simulink model "hcu_main_dspace"  (Simulink 8.2)
settings: Solver=FixedStepDiscrete  StartTime=0.0  StopTime=Inf  FixedStep=0.005  RelTol=1e-3
PostLoadFcn:
  | , if any(exist('dsrtsu_mdlpostloadfcn', 'file') == [2, 3, 6]), try dsrtsu_mdlpostloadfcn('Execute', bdroot); catch fprintf('Error in PostLoadFcn (dsrtsu_mdlpostloadfcn) for model "%s":\n %s\n', bdroot, lasterr); end, end,
values from neighbouring files (symbols this model uses):
  C_TASK_5MS_S = (	C_TICK_TIME_S      	)    [hcu_local_hdr.m]
  ENUM_GEARPOSN_1ST = uint8(  1  )    [hcu_local_hdr.m]
  ENUM_GEARPOSN_2ND = uint8(  2  )    [hcu_local_hdr.m]
  ENUM_GEARPOSN_3RD = uint8(  3  )    [hcu_local_hdr.m]
  ENUM_GEARPOSN_4TH = uint8(  4  )    [hcu_local_hdr.m]
  ENUM_GEARPOSN_5TH = uint8(  5  )    [hcu_local_hdr.m]
  ENUM_GEARPOSN_6TH = uint8(  6  )    [hcu_local_hdr.m]
  ENUM_GEARPOSN_R = uint8(  7  )    [hcu_local_hdr.m]
undefined symbols (not defined in the file or in its folder): rticanmm_blockfcn, rticanmm_initfcn
libraries: rtimmsu_dsrtlib x3, simulink x2, hal x2, app x1, rtiethernetudplib x1, inp x1, outp x1, hcu_lib x1
(part 2 of 4)

== system hcu_main_dspace/RTICANMM MainBlock1 ==
  TXData : Inport
  ModelClose : Subsystem  mask(RTICANMMModelClose){}
  TRC Exclusion : rtimmsu_dsrtlib/TRC Exclusion
  TXINselector1 : BusSelector  OutputSignals=ADAS1.ADAS1_Checksum,ADAS1.ADAS1_LifeCount,ADAS1.ADAS_StrTqReq_A,ADAS1.ADAS_StrAngReq_A,ADAS1.ADAS_EPSMode,ADAS1.ADAS_StrTqReqProt,ADAS1.ADAS_StrTqReq,ADAS1.ADAS_StrAngReqProt,ADAS1.ADAS_StrAngReq,ADAS2.ADAS2_Checksum,ADAS2.ADAS2_LifeCount,ADAS2.ADAS_VehHoldReq,ADAS2.ADAS_BrakePrefillReq_A,ADAS2.ADAS_BrakePrefillReq,ADAS2.ADAS_AEBReq_A,ADAS2.ADAS_AEBReq,ADAS2.ADAS_ForceIdle_A,ADAS2.ADAS_DecReq_Prot,ADAS2.ADAS_DecReq,ADAS2.ADAS_DecReq_A,ADAS2.ADAS_TqReq_A,ADAS2.ADAS_ForceIdle,ADAS2.ADAS_TqReqProt,ADAS2.ADAS_TqReq,ADAS3.ADAS3_Checksum,ADAS3.ADAS3_LifeCount,ADAS3.ForceLowBeam,ADAS3.LeftTurnLightReq,ADAS3.RightTurnLightReq,ADAS3.HazardWarningReq,ADAS3.ADAS_MIL,ADAS3.RampDownEnable,ADAS3.RampDownTime,ADAS3.ADAS_ShftPosnReq_A,ADAS3.ADAS_ShftPosnReq,ADAS3.ADAS_VehSpdLim_A,ADAS3.ADAS_GearPosnReq_A,ADAS3.ADAS_GearPosnReq,ADAS3.ADAS_VehSpdLim,ADAS4.ADASFaultWarningReq,ADAS4.HapticWarningReq,ADAS4.ADAS_APSEnable,ADAS4.ADAS_PilotMode,ADAS4.ADAS_IGSAStatus,ADAS4.ADAS_LFCMode,ADAS4.ADAS_MAPPStatus,ADAS4.ADAS_MAPAStatus,ADAS4.ADAS_LCSStatus,ADAS4.ADAS_LFCStatus,ADAS4.ADAS_LKAStatus,ADAS4.ADAS_ACCStatus,ADAS4.ADAS_FCWStatus,ADAS4.ADAS_AEBStatus,ADAS4.MAPPHMIWarningReq,ADAS4.MAPAHMIWarningReq,ADAS4.LCSHMIWarningReq,ADAS4.LFCHMIWarningReq,ADAS4.LKAHMIWarningReq,ADAS4.IGSAHMIWarningReq,ADAS4.AEBHMIWarningReq,ADAS4.ACCHMIWarningReq,ADAS4.FCWHMIWarningReq,ADAS5.ADAS_FaultMode,ADAS5.ADAS_LaneModeR,ADAS5.ADAS_LaneModeL,ADAS5.SeleTimeGapLvl,ADAS5.SetTimeGapLvl,ADAS5.IGSASetSpeed,ADAS5.ACCSetSpeed,ADAS5.SetVehTimeGap,ADAS5.LeadVehTimeGap,ADAS5.TargetType
  converter : Subsystem  mask(CANnedyVector2Bus){}
      mask help: Do not change.
      mask Display: disp('Vector to\nBus')
  sfcn : S-Function  InitFcn=rticanmm_initfcn(gcb, 'SFCNs')  FunctionName=RTICANMM_MAIN_CAN_1  EnableBusSupport=off
      mask init:
      | rticanmm_initfcn(gcb, 'SFCNs')
  RX_Data : Outport
  wires:
  TXData/1 -> TXINselector1/1
  TXINselector1/1 -> sfcn/1  "<ADAS1_Checksum>"
  TXINselector1/2 -> sfcn/2  "<ADAS1_LifeCount>"
  TXINselector1/3 -> sfcn/3  "<ADAS_StrTqReq_A>"
  TXINselector1/4 -> sfcn/4  "<ADAS_StrAngReq_A>"
  TXINselector1/5 -> sfcn/5  "<ADAS_EPSMode>"
  TXINselector1/6 -> sfcn/6  "<ADAS_StrTqReqProt>"
  TXINselector1/7 -> sfcn/7  "<ADAS_StrTqReq>"
  TXINselector1/8 -> sfcn/8  "<ADAS_StrAngReqProt>"
  TXINselector1/9 -> sfcn/9  "<ADAS_StrAngReq>"
  TXINselector1/10 -> sfcn/10  "<ADAS2_Checksum>"
  TXINselector1/11 -> sfcn/11  "<ADAS2_LifeCount>"
  TXINselector1/12 -> sfcn/12  "<ADAS_VehHoldReq>"
  TXINselector1/13 -> sfcn/13  "<ADAS_BrakePrefillReq_A>"
  TXINselector1/14 -> sfcn/14  "<ADAS_BrakePrefillReq>"
  TXINselector1/15 -> sfcn/15  "<ADAS_AEBReq_A>"
  TXINselector1/16 -> sfcn/16  "<ADAS_AEBReq>"
  TXINselector1/17 -> sfcn/17  "<ADAS_ForceIdle_A>"
  TXINselector1/18 -> sfcn/18  "<ADAS_DecReq_Prot>"
  TXINselector1/19 -> sfcn/19  "<ADAS_DecReq>"
  TXINselector1/20 -> sfcn/20  "<ADAS_DecReq_A>"
  TXINselector1/21 -> sfcn/21  "<ADAS_TqReq_A>"
  TXINselector1/22 -> sfcn/22  "<ADAS_ForceIdle>"
  TXINselector1/23 -> sfcn/23  "<ADAS_TqReqProt>"
  TXINselector1/24 -> sfcn/24  "<ADAS_TqReq>"
  TXINselector1/25 -> sfcn/25  "<ADAS3_Checksum>"
  TXINselector1/26 -> sfcn/26  "<ADAS3_LifeCount>"
  TXINselector1/27 -> sfcn/27  "<ForceLowBeam>"
  TXINselector1/28 -> sfcn/28  "<LeftTurnLightReq>"
  TXINselector1/29 -> sfcn/29  "<RightTurnLightReq>"
  TXINselector1/30 -> sfcn/30  "<HazardWarningReq>"
  TXINselector1/31 -> sfcn/31  "<ADAS_MIL>"
  TXINselector1/32 -> sfcn/32  "<RampDownEnable>"
  TXINselector1/33 -> sfcn/33  "<RampDownTime>"
  TXINselector1/34 -> sfcn/34  "<ADAS_ShftPosnReq_A>"
  TXINselector1/35 -> sfcn/35  "<ADAS_ShftPosnReq>"
  TXINselector1/36 -> sfcn/36  "<ADAS_VehSpdLim_A>"
  TXINselector1/37 -> sfcn/37  "<ADAS_GearPosnReq_A>"
  TXINselector1/38 -> sfcn/38  "<ADAS_GearPosnReq>"
  TXINselector1/39 -> sfcn/39  "<ADAS_VehSpdLim>"
  TXINselector1/40 -> sfcn/40  "<ADASFaultWarningReq>"
  TXINselector1/41 -> sfcn/41  "<HapticWarningReq>"
  TXINselector1/42 -> sfcn/42  "<ADAS_APSEnable>"
  TXINselector1/43 -> sfcn/43  "<ADAS_PilotMode>"
  TXINselector1/44 -> sfcn/44  "<ADAS_IGSAStatus>"
  TXINselector1/45 -> sfcn/45  "<ADAS_LFCMode>"
  TXINselector1/46 -> sfcn/46  "<ADAS_MAPPStatus>"
  TXINselector1/47 -> sfcn/47  "<ADAS_MAPAStatus>"
  TXINselector1/48 -> sfcn/48  "<ADAS_LCSStatus>"
  TXINselector1/49 -> sfcn/49  "<ADAS_LFCStatus>"
  TXINselector1/50 -> sfcn/50  "<ADAS_LKAStatus>"
  TXINselector1/51 -> sfcn/51  "<ADAS_ACCStatus>"
  TXINselector1/52 -> sfcn/52  "<ADAS_FCWStatus>"
  TXINselector1/53 -> sfcn/53  "<ADAS_AEBStatus>"
  TXINselector1/54 -> sfcn/54  "<MAPPHMIWarningReq>"
  TXINselector1/55 -> sfcn/55  "<MAPAHMIWarningReq>"
  TXINselector1/56 -> sfcn/56  "<LCSHMIWarningReq>"
  TXINselector1/57 -> sfcn/57  "<LFCHMIWarningReq>"
  TXINselector1/58 -> sfcn/58  "<LKAHMIWarningReq>"
  TXINselector1/59 -> sfcn/59  "<IGSAHMIWarningReq>"
  TXINselector1/60 -> sfcn/60  "<AEBHMIWarningReq>"
  TXINselector1/61 -> sfcn/61  "<ACCHMIWarningReq>"
  TXINselector1/62 -> sfcn/62  "<FCWHMIWarningReq>"
  TXINselector1/63 -> sfcn/63  "<ADAS_FaultMode>"
  TXINselector1/64 -> sfcn/64  "<ADAS_LaneModeR>"
  TXINselector1/65 -> sfcn/65  "<ADAS_LaneModeL>"
  TXINselector1/66 -> sfcn/66  "<SeleTimeGapLvl>"
  TXINselector1/67 -> sfcn/67  "<SetTimeGapLvl>"
  TXINselector1/68 -> sfcn/68  "<IGSASetSpeed>"
  TXINselector1/69 -> sfcn/69  "<ACCSetSpeed>"
  TXINselector1/70 -> sfcn/70  "<SetVehTimeGap>"
  TXINselector1/71 -> sfcn/71  "<LeadVehTimeGap>"
  TXINselector1/72 -> sfcn/72  "<TargetType>"
  converter/1(out) -> RX_Data/1
  sfcn/1 -> converter/1(in_1)
  sfcn/2 -> converter/2(in_2)
  sfcn/3 -> converter/3(in_3)
  sfcn/4 -> converter/4(in_4)
  sfcn/5 -> converter/5(in_5)
  sfcn/6 -> converter/6(in_6)
  sfcn/7 -> converter/7(in_7)
  sfcn/8 -> converter/8(in_8)
  sfcn/9 -> converter/9(in_9)
  sfcn/10 -> converter/10(in_10)
  sfcn/11 -> converter/11(in_11)
  sfcn/12 -> converter/12(in_12)
  sfcn/13 -> converter/13(in_13)
  sfcn/14 -> converter/14(in_14)
  sfcn/15 -> converter/15(in_15)
  sfcn/16 -> converter/16(in_16)
  sfcn/17 -> converter/17(in_17)
  sfcn/18 -> converter/18(in_18)
  sfcn/19 -> converter/19(in_19)
  sfcn/20 -> converter/20(in_20)
  sfcn/21 -> converter/21(in_21)
  sfcn/22 -> converter/22(in_22)
  sfcn/23 -> converter/23(in_23)
  sfcn/24 -> converter/24(in_24)
  sfcn/25 -> converter/25(in_25)
  sfcn/26 -> converter/26(in_26)
  sfcn/27 -> converter/27(in_27)
  sfcn/28 -> converter/28(in_28)
  sfcn/29 -> converter/29(in_29)
  sfcn/30 -> converter/30(in_30)
  sfcn/31 -> converter/31(in_31)
  sfcn/32 -> converter/32(in_32)
  sfcn/33 -> converter/33(in_33)
  sfcn/34 -> converter/34(in_34)
  sfcn/35 -> converter/35(in_35)
  sfcn/36 -> converter/36(in_36)
  sfcn/37 -> converter/37(in_37)
  sfcn/38 -> converter/38(in_38)
  sfcn/39 -> converter/39(in_39)
  sfcn/40 -> converter/40(in_40)
  sfcn/41 -> converter/41(in_41)
  sfcn/42 -> converter/42(in_42)
  sfcn/43 -> converter/43(in_43)
  sfcn/44 -> converter/44(in_44)
  sfcn/45 -> converter/45(in_45)
  sfcn/46 -> converter/46(in_46)
  sfcn/47 -> converter/47(in_47)
  sfcn/48 -> converter/48(in_48)
  sfcn/49 -> converter/49(in_49)
  sfcn/50 -> converter/50(in_50)
  sfcn/51 -> converter/51(in_51)
  sfcn/52 -> converter/52(in_52)
  sfcn/53 -> converter/53(in_53)
  sfcn/54 -> converter/54(in_54)
  sfcn/55 -> converter/55(in_55)
  sfcn/56 -> converter/56(in_56)
  sfcn/57 -> converter/57(in_57)
  sfcn/58 -> converter/58(in_58)
  sfcn/59 -> converter/59(in_59)
  sfcn/60 -> converter/60(in_60)
  sfcn/61 -> converter/61(in_61)
  sfcn/62 -> converter/62(in_62)
  sfcn/63 -> converter/63(in_63)
  sfcn/64 -> converter/64(in_64)
  sfcn/65 -> converter/65(in_65)
  sfcn/66 -> converter/66(in_66)
  sfcn/67 -> converter/67(in_67)
  sfcn/68 -> converter/68(in_68)
  sfcn/69 -> converter/69(in_69)
  sfcn/70 -> converter/70(in_70)
  sfcn/71 -> converter/71(in_71)
  sfcn/72 -> converter/72(in_72)
  sfcn/73 -> converter/73(in_73)
  sfcn/74 -> converter/74(in_74)
  sfcn/75 -> converter/75(in_75)
  sfcn/76 -> converter/76(in_76)
  sfcn/77 -> converter/77(in_77)
  sfcn/78 -> converter/78(in_78)
  sfcn/79 -> converter/79(in_79)
  sfcn/80 -> converter/80(in_80)
  sfcn/81 -> converter/81(in_81)
  sfcn/82 -> converter/82(in_82)
  sfcn/83 -> converter/83(in_83)
  sfcn/84 -> converter/84(in_84)
  sfcn/85 -> converter/85(in_85)
  sfcn/86 -> converter/86(in_86)
  sfcn/87 -> converter/87(in_87)
  sfcn/88 -> converter/88(in_88)
  sfcn/89 -> converter/89(in_89)
  sfcn/90 -> converter/90(in_90)
  sfcn/91 -> converter/91(in_91)
  sfcn/92 -> converter/92(in_92)
  sfcn/93 -> converter/93(in_93)
  sfcn/94 -> converter/94(in_94)
  sfcn/95 -> converter/95(in_95)
  sfcn/96 -> converter/96(in_96)
  sfcn/97 -> converter/97(in_97)
  sfcn/98 -> converter/98(in_98)
  sfcn/99 -> converter/99(in_99)
  sfcn/100 -> converter/100(in_100)
  sfcn/101 -> converter/101(in_101)
  sfcn/102 -> converter/102(in_102)
  sfcn/103 -> converter/103(in_103)
  sfcn/104 -> converter/104(in_104)
  sfcn/105 -> converter/105(in_105)
  sfcn/106 -> converter/106(in_106)
  sfcn/107 -> converter/107(in_107)
  sfcn/108 -> converter/108(in_108)
  sfcn/109 -> converter/109(in_109)
  sfcn/110 -> converter/110(in_110)
  sfcn/111 -> converter/111(in_111)
  sfcn/112 -> converter/112(in_112)
  sfcn/113 -> converter/113(in_113)
  sfcn/114 -> converter/114(in_114)
  sfcn/115 -> converter/115(in_115)
  sfcn/116 -> converter/116(in_116)
  sfcn/117 -> converter/117(in_117)
  sfcn/118 -> converter/118(in_118)
  sfcn/119 -> converter/119(in_119)
  sfcn/120 -> converter/120(in_120)
  sfcn/121 -> converter/121(in_121)
  sfcn/122 -> converter/122(in_122)
  sfcn/123 -> converter/123(in_123)
  sfcn/124 -> converter/124(in_124)
  sfcn/125 -> converter/125(in_125)
  sfcn/126 -> converter/126(in_126)
  sfcn/127 -> converter/127(in_127)
  sfcn/128 -> converter/128(in_128)
  sfcn/129 -> converter/129(in_129)
  sfcn/130 -> converter/130(in_130)
  sfcn/131 -> converter/131(in_131)
  sfcn/132 -> converter/132(in_132)
  sfcn/133 -> converter/133(in_133)
  sfcn/134 -> converter/134(in_134)
  sfcn/135 -> converter/135(in_135)
  sfcn/136 -> converter/136(in_136)
  sfcn/137 -> converter/137(in_137)
  sfcn/138 -> converter/138(in_138)
  sfcn/139 -> converter/139(in_139)
  sfcn/140 -> converter/140(in_140)
  sfcn/141 -> converter/141(in_141)
  sfcn/142 -> converter/142(in_142)
  sfcn/143 -> converter/143(in_143)
  sfcn/144 -> converter/144(in_144)
  sfcn/145 -> converter/145(in_145)
  sfcn/146 -> converter/146(in_146)
  sfcn/147 -> converter/147(in_147)
  sfcn/148 -> converter/148(in_148)
  sfcn/149 -> converter/149(in_149)
  sfcn/150 -> converter/150(in_150)
  sfcn/151 -> converter/151(in_151)
  sfcn/152 -> converter/152(in_152)
  sfcn/153 -> converter/153(in_153)
  sfcn/154 -> converter/154(in_154)
  sfcn/155 -> converter/155(in_155)
  sfcn/156 -> converter/156(in_156)
  sfcn/157 -> converter/157(in_157)
  sfcn/158 -> converter/158(in_158)
  sfcn/159 -> converter/159(in_159)
  sfcn/160 -> converter/160(in_160)
  sfcn/161 -> converter/161(in_161)
  sfcn/162 -> converter/162(in_162)
  sfcn/163 -> converter/163(in_163)
  sfcn/164 -> converter/164(in_164)
  sfcn/165 -> converter/165(in_165)
  sfcn/166 -> converter/166(in_166)
  sfcn/167 -> converter/167(in_167)
  sfcn/168 -> converter/168(in_168)
  sfcn/169 -> converter/169(in_169)
  sfcn/170 -> converter/170(in_170)
  sfcn/171 -> converter/171(in_171)
  sfcn/172 -> converter/172(in_172)
  sfcn/173 -> converter/173(in_173)
  sfcn/174 -> converter/174(in_174)
  sfcn/175 -> converter/175(in_175)
  sfcn/176 -> converter/176(in_176)
  sfcn/177 -> converter/177(in_177)
  sfcn/178 -> converter/178(in_178)
  sfcn/179 -> converter/179(in_179)
  sfcn/180 -> converter/180(in_180)
  sfcn/181 -> converter/181(in_181)
  sfcn/182 -> converter/182(in_182)
  sfcn/183 -> converter/183(in_183)
  sfcn/184 -> converter/184(in_184)
  sfcn/185 -> converter/185(in_185)
  sfcn/186 -> converter/186(in_186)
  sfcn/187 -> converter/187(in_187)
  sfcn/188 -> converter/188(in_188)
  sfcn/189 -> converter/189(in_189)
  sfcn/190 -> converter/190(in_190)
  sfcn/191 -> converter/191(in_191)
  sfcn/192 -> converter/192(in_192)
  sfcn/193 -> converter/193(in_193)
  sfcn/194 -> converter/194(in_194)
  sfcn/195 -> converter/195(in_195)
  sfcn/196 -> converter/196(in_196)
  sfcn/197 -> converter/197(in_197)
  sfcn/198 -> converter/198(in_198)
  sfcn/199 -> converter/199(in_199)
  sfcn/200 -> converter/200(in_200)
  sfcn/201 -> converter/201(in_201)
  sfcn/202 -> converter/202(in_202)
  sfcn/203 -> converter/203(in_203)
  sfcn/204 -> converter/204(in_204)
  sfcn/205 -> converter/205(in_205)
  sfcn/206 -> converter/206(in_206)
  sfcn/207 -> converter/207(in_207)
  sfcn/208 -> converter/208(in_208)
  sfcn/209 -> converter/209(in_209)
  sfcn/210 -> converter/210(in_210)
  sfcn/211 -> converter/211(in_211)
  sfcn/212 -> converter/212(in_212)
  sfcn/213 -> converter/213(in_213)
  sfcn/214 -> converter/214(in_214)
  sfcn/215 -> converter/215(in_215)
  sfcn/216 -> converter/216(in_216)
  sfcn/217 -> converter/217(in_217)
  sfcn/218 -> converter/218(in_218)
  sfcn/219 -> converter/219(in_219)
  sfcn/220 -> converter/220(in_220)
  sfcn/221 -> converter/221(in_221)
  sfcn/222 -> converter/222(in_222)
  sfcn/223 -> converter/223(in_223)
  sfcn/224 -> converter/224(in_224)
  sfcn/225 -> converter/225(in_225)
  sfcn/226 -> converter/226(in_226)
  sfcn/227 -> converter/227(in_227)
  sfcn/228 -> converter/228(in_228)
  sfcn/229 -> converter/229(in_229)
  sfcn/230 -> converter/230(in_230)
  sfcn/231 -> converter/231(in_231)
  sfcn/232 -> converter/232(in_232)
  sfcn/233 -> converter/233(in_233)
  sfcn/234 -> converter/234(in_234)
  sfcn/235 -> converter/235(in_235)
  sfcn/236 -> converter/236(in_236)
  sfcn/237 -> converter/237(in_237)
  sfcn/238 -> converter/238(in_238)
  sfcn/239 -> converter/239(in_239)
  sfcn/240 -> converter/240(in_240)
  sfcn/241 -> converter/241(in_241)
  sfcn/242 -> converter/242(in_242)
  sfcn/243 -> converter/243(in_243)
  sfcn/244 -> converter/244(in_244)
  sfcn/245 -> converter/245(in_245)
  sfcn/246 -> converter/246(in_246)
  sfcn/247 -> converter/247(in_247)
  sfcn/248 -> converter/248(in_248)
  sfcn/249 -> converter/249(in_249)
  sfcn/250 -> converter/250(in_250)
  sfcn/251 -> converter/251(in_251)
  sfcn/252 -> converter/252(in_252)
  sfcn/253 -> converter/253(in_253)
  sfcn/254 -> converter/254(in_254)
  sfcn/255 -> converter/255(in_255)
  sfcn/256 -> converter/256(in_256)
  sfcn/257 -> converter/257(in_257)
  sfcn/258 -> converter/258(in_258)
  sfcn/259 -> converter/259(in_259)
  sfcn/260 -> converter/260(in_260)
  sfcn/261 -> converter/261(in_261)
  sfcn/262 -> converter/262(in_262)
  sfcn/263 -> converter/263(in_263)
  sfcn/264 -> converter/264(in_264)
  sfcn/265 -> converter/265(in_265)
  sfcn/266 -> converter/266(in_266)
  sfcn/267 -> converter/267(in_267)
  sfcn/268 -> converter/268(in_268)
  sfcn/269 -> converter/269(in_269)
  sfcn/270 -> converter/270(in_270)
  sfcn/271 -> converter/271(in_271)
  sfcn/272 -> converter/272(in_272)
  sfcn/273 -> converter/273(in_273)
  sfcn/274 -> converter/274(in_274)
  sfcn/275 -> converter/275(in_275)
  sfcn/276 -> converter/276(in_276)
  sfcn/277 -> converter/277(in_277)
  sfcn/278 -> converter/278(in_278)
  sfcn/279 -> converter/279(in_279)
  sfcn/280 -> converter/280(in_280)
  sfcn/281 -> converter/281(in_281)
  sfcn/282 -> converter/282(in_282)
  sfcn/283 -> converter/283(in_283)
  sfcn/284 -> converter/284(in_284)
  sfcn/285 -> converter/285(in_285)
  sfcn/286 -> converter/286(in_286)
  sfcn/287 -> converter/287(in_287)
  sfcn/288 -> converter/288(in_288)
  sfcn/289 -> converter/289(in_289)
  sfcn/290 -> converter/290(in_290)
  sfcn/291 -> converter/291(in_291)
  sfcn/292 -> converter/292(in_292)
  sfcn/293 -> converter/293(in_293)
  sfcn/294 -> converter/294(in_294)
  sfcn/295 -> converter/295(in_295)
  sfcn/296 -> converter/296(in_296)
  sfcn/297 -> converter/297(in_297)
  sfcn/298 -> converter/298(in_298)
  sfcn/299 -> converter/299(in_299)
  sfcn/300 -> converter/300(in_300)
  sfcn/301 -> converter/301(in_301)
  sfcn/302 -> converter/302(in_302)
  sfcn/303 -> converter/303(in_303)
  sfcn/304 -> converter/304(in_304)
  sfcn/305 -> converter/305(in_305)
  sfcn/306 -> converter/306(in_306)
  sfcn/307 -> converter/307(in_307)
  sfcn/308 -> converter/308(in_308)
  sfcn/309 -> converter/309(in_309)
  sfcn/310 -> converter/310(in_310)
  sfcn/311 -> converter/311(in_311)
  sfcn/312 -> converter/312(in_312)
  sfcn/313 -> converter/313(in_313)
  sfcn/314 -> converter/314(in_314)
  sfcn/315 -> converter/315(in_315)
  sfcn/316 -> converter/316(in_316)
  sfcn/317 -> converter/317(in_317)
  sfcn/318 -> converter/318(in_318)
  sfcn/319 -> converter/319(in_319)
  sfcn/320 -> converter/320(in_320)
  sfcn/321 -> converter/321(in_321)
  sfcn/322 -> converter/322(in_322)
  sfcn/323 -> converter/323(in_323)
  sfcn/324 -> converter/324(in_324)
  sfcn/325 -> converter/325(in_325)
  sfcn/326 -> converter/326(in_326)
  sfcn/327 -> converter/327(in_327)
  sfcn/328 -> converter/328(in_328)
  sfcn/329 -> converter/329(in_329)
  sfcn/330 -> converter/330(in_330)
  sfcn/331 -> converter/331(in_331)
  sfcn/332 -> converter/332(in_332)
  sfcn/333 -> converter/333(in_333)
  sfcn/334 -> converter/334(in_334)
  sfcn/335 -> converter/335(in_335)
  sfcn/336 -> converter/336(in_336)
  sfcn/337 -> converter/337(in_337)
  sfcn/338 -> converter/338(in_338)
  sfcn/339 -> converter/339(in_339)
  sfcn/340 -> converter/340(in_340)
  sfcn/341 -> converter/341(in_341)
  sfcn/342 -> converter/342(in_342)
  sfcn/343 -> converter/343(in_343)
  sfcn/344 -> converter/344(in_344)
  sfcn/345 -> converter/345(in_345)
  sfcn/346 -> converter/346(in_346)
  sfcn/347 -> converter/347(in_347)
  sfcn/348 -> converter/348(in_348)
  sfcn/349 -> converter/349(in_349)
  sfcn/350 -> converter/350(in_350)
  sfcn/351 -> converter/351(in_351)
  sfcn/352 -> converter/352(in_352)
  sfcn/353 -> converter/353(in_353)
  sfcn/354 -> converter/354(in_354)
  sfcn/355 -> converter/355(in_355)
  sfcn/356 -> converter/356(in_356)
  sfcn/357 -> converter/357(in_357)
  sfcn/358 -> converter/358(in_358)
  sfcn/359 -> converter/359(in_359)
  sfcn/360 -> converter/360(in_360)
  sfcn/361 -> converter/361(in_361)
  sfcn/362 -> converter/362(in_362)
  sfcn/363 -> converter/363(in_363)
  sfcn/364 -> converter/364(in_364)
  sfcn/365 -> converter/365(in_365)
  sfcn/366 -> converter/366(in_366)
  sfcn/367 -> converter/367(in_367)
  sfcn/368 -> converter/368(in_368)
  sfcn/369 -> converter/369(in_369)
  sfcn/370 -> converter/370(in_370)
  sfcn/371 -> converter/371(in_371)
  sfcn/372 -> converter/372(in_372)
  sfcn/373 -> converter/373(in_373)
  sfcn/374 -> converter/374(in_374)
  sfcn/375 -> converter/375(in_375)
  sfcn/376 -> converter/376(in_376)
  sfcn/377 -> converter/377(in_377)
  sfcn/378 -> converter/378(in_378)
  sfcn/379 -> converter/379(in_379)
  sfcn/380 -> converter/380(in_380)
  sfcn/381 -> converter/381(in_381)
  sfcn/382 -> converter/382(in_382)
  sfcn/383 -> converter/383(in_383)
  sfcn/384 -> converter/384(in_384)
  sfcn/385 -> converter/385(in_385)
  sfcn/386 -> converter/386(in_386)
  sfcn/387 -> converter/387(in_387)
  sfcn/388 -> converter/388(in_388)
  sfcn/389 -> converter/389(in_389)
  sfcn/390 -> converter/390(in_390)
  sfcn/391 -> converter/391(in_391)
  sfcn/392 -> converter/392(in_392)
  sfcn/393 -> converter/393(in_393)
  sfcn/394 -> converter/394(in_394)
  sfcn/395 -> converter/395(in_395)
  sfcn/396 -> converter/396(in_396)
  sfcn/397 -> converter/397(in_397)
  sfcn/398 -> converter/398(in_398)
  sfcn/399 -> converter/399(in_399)
  sfcn/400 -> converter/400(in_400)
  sfcn/401 -> converter/401(in_401)
  sfcn/402 -> converter/402(in_402)
  sfcn/403 -> converter/403(in_403)
  sfcn/404 -> converter/404(in_404)
  sfcn/405 -> converter/405(in_405)
  sfcn/406 -> converter/406(in_406)
  sfcn/407 -> converter/407(in_407)
  sfcn/408 -> converter/408(in_408)
  sfcn/409 -> converter/409(in_409)
  sfcn/410 -> converter/410(in_410)
  sfcn/411 -> converter/411(in_411)
  sfcn/412 -> converter/412(in_412)
  sfcn/413 -> converter/413(in_413)
  sfcn/414 -> converter/414(in_414)
  sfcn/415 -> converter/415(in_415)
  sfcn/416 -> converter/416(in_416)
  sfcn/417 -> converter/417(in_417)
  sfcn/418 -> converter/418(in_418)
  sfcn/419 -> converter/419(in_419)
  sfcn/420 -> converter/420(in_420)
  sfcn/421 -> converter/421(in_421)
  sfcn/422 -> converter/422(in_422)
  sfcn/423 -> converter/423(in_423)
  sfcn/424 -> converter/424(in_424)
  sfcn/425 -> converter/425(in_425)
  sfcn/426 -> converter/426(in_426)
  sfcn/427 -> converter/427(in_427)
  sfcn/428 -> converter/428(in_428)
  sfcn/429 -> converter/429(in_429)
  sfcn/430 -> converter/430(in_430)
  sfcn/431 -> converter/431(in_431)
  sfcn/432 -> converter/432(in_432)
  sfcn/433 -> converter/433(in_433)
  sfcn/434 -> converter/434(in_434)
  sfcn/435 -> converter/435(in_435)
  sfcn/436 -> converter/436(in_436)
  sfcn/437 -> converter/437(in_437)
  sfcn/438 -> converter/438(in_438)
  sfcn/439 -> converter/439(in_439)
  sfcn/440 -> converter/440(in_440)
  sfcn/441 -> converter/441(in_441)
  sfcn/442 -> converter/442(in_442)
  sfcn/443 -> converter/443(in_443)
  sfcn/444 -> converter/444(in_444)
  sfcn/445 -> converter/445(in_445)
  sfcn/446 -> converter/446(in_446)
  sfcn/447 -> converter/447(in_447)
  sfcn/448 -> converter/448(in_448)
  sfcn/449 -> converter/449(in_449)
  sfcn/450 -> converter/450(in_450)
  sfcn/451 -> converter/451(in_451)
  sfcn/452 -> converter/452(in_452)
  sfcn/453 -> converter/453(in_453)
  sfcn/454 -> converter/454(in_454)
  sfcn/455 -> converter/455(in_455)
  sfcn/456 -> converter/456(in_456)
  sfcn/457 -> converter/457(in_457)
  sfcn/458 -> converter/458(in_458)
  sfcn/459 -> converter/459(in_459)
  sfcn/460 -> converter/460(in_460)
  sfcn/461 -> converter/461(in_461)
  sfcn/462 -> converter/462(in_462)
  sfcn/463 -> converter/463(in_463)
  sfcn/464 -> converter/464(in_464)
  sfcn/465 -> converter/465(in_465)
  sfcn/466 -> converter/466(in_466)
  sfcn/467 -> converter/467(in_467)
  sfcn/468 -> converter/468(in_468)
  sfcn/469 -> converter/469(in_469)
  sfcn/470 -> converter/470(in_470)
  sfcn/471 -> converter/471(in_471)
  sfcn/472 -> converter/472(in_472)
  sfcn/473 -> converter/473(in_473)
  sfcn/474 -> converter/474(in_474)
  sfcn/475 -> converter/475(in_475)
  sfcn/476 -> converter/476(in_476)
  sfcn/477 -> converter/477(in_477)
  sfcn/478 -> converter/478(in_478)
  sfcn/479 -> converter/479(in_479)
  sfcn/480 -> converter/480(in_480)
  sfcn/481 -> converter/481(in_481)
  sfcn/482 -> converter/482(in_482)
  sfcn/483 -> converter/483(in_483)
  sfcn/484 -> converter/484(in_484)
  sfcn/485 -> converter/485(in_485)

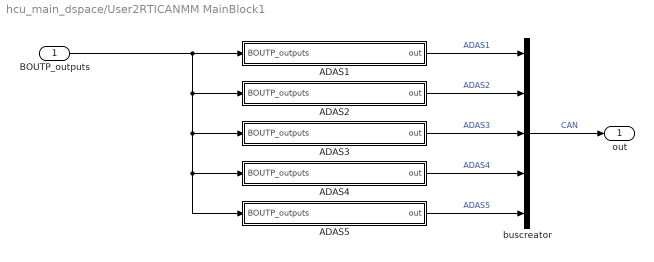
== system hcu_main_dspace/User2RTICANMM MainBlock1 ==
  BOUTP_outputs : Inport  OutDataTypeStr=Bus: BOUTP_outputs
  ADAS1 : Subsystem
  ADAS2 : Subsystem
  ADAS3 : Subsystem
  ADAS4 : Subsystem
  ADAS5 : Subsystem
  buscreator : BusCreator  Inputs=5
  out : Outport
  wires:
  ADAS1/1(out) -> buscreator/1  "ADAS1"
  ADAS2/1(out) -> buscreator/2  "ADAS2"
  ADAS3/1(out) -> buscreator/3  "ADAS3"
  ADAS4/1(out) -> buscreator/4  "ADAS4"
  ADAS5/1(out) -> buscreator/5  "ADAS5"
  buscreator/1 -> out/1  "CAN"
  BOUTP_outputs/1 -> ADAS2/1(BOUTP_outputs), ADAS3/1(BOUTP_outputs), ADAS5/1(BOUTP_outputs), ADAS4/1(BOUTP_outputs), ADAS1/1(BOUTP_outputs)

== system hcu_main_dspace/User2RTICANMM MainBlock_ ==
  CAN1_Rx : Inport
  ABS2_C : Subsystem
  ABS4_C : Subsystem
  SAS1 : Subsystem
  SpeedInformation : Subsystem
  YawRateInformation : Subsystem
  buscreator : BusCreator  Inputs=5
  out : Outport
  wires:
  ABS2_C/1(out) -> buscreator/1  "ABS2_C"
  ABS4_C/1(out) -> buscreator/2  "ABS4_C"
  SAS1/1(out) -> buscreator/3  "SAS1"
  SpeedInformation/1(out) -> buscreator/4  "SpeedInformation"
  YawRateInformation/1(out) -> buscreator/5  "YawRateInformation"
  buscreator/1 -> out/1  "CAN"
  CAN1_Rx/1 -> YawRateInformation/1(CAN1_Rx), SpeedInformation/1(CAN1_Rx), SAS1/1(CAN1_Rx), ABS4_C/1(CAN1_Rx), ABS2_C/1(CAN1_Rx1)

== system hcu_main_dspace/RTI Data/RTI Data Store ==
  RTI Data Store : Subsystem  mask(RTI_DATA_STORE){}
      mask help:
      | RTI Data Store Block. This block is used by RTI to store internal model dependent data. Deleting this block will result in data loss.
      |
      | NEVER DELETE, COPY, OR MODIFY THIS BLOCK!
      mask Help:
      | RTI Data Store Block. This block is used by RTI to store internal model dependent data. Deleting this block will result in data loss.
      | 
      | NEVER DELETE, COPY, OR MODIFY THIS BLOCK!
      mask Display: text(0.5, 0.5, ' ', 'HorizontalAlignment', 'center');

== system hcu_main_dspace/RTICANMM ControllerSetup/ModelClose ==

== system hcu_main_dspace/RTICANMM ControllerSetup1/ModelClose ==

== system hcu_main_dspace/RTICANMM GeneralSetup/ModelClose ==

== system hcu_main_dspace/RTICANMM MainBlock/ModelClose ==
